simulink model "stuSimulation"  (R2019b)
settings: Solver=VariableStepAuto  StartTime=0.0  StopTime=0.1  RelTol=1e-3
undefined symbols (not defined in the file): doppler
libraries: commchan3 x2, dspsrcs4 x2, dsparch4 x1
settings Model: Creator=dm  LastModifiedBy=LYM
settings DebuggingCC: SFMachineParentedDataDiag=error
settings GRTTargetCC: RTWCAPISignals=on  RTWCAPIParams=on

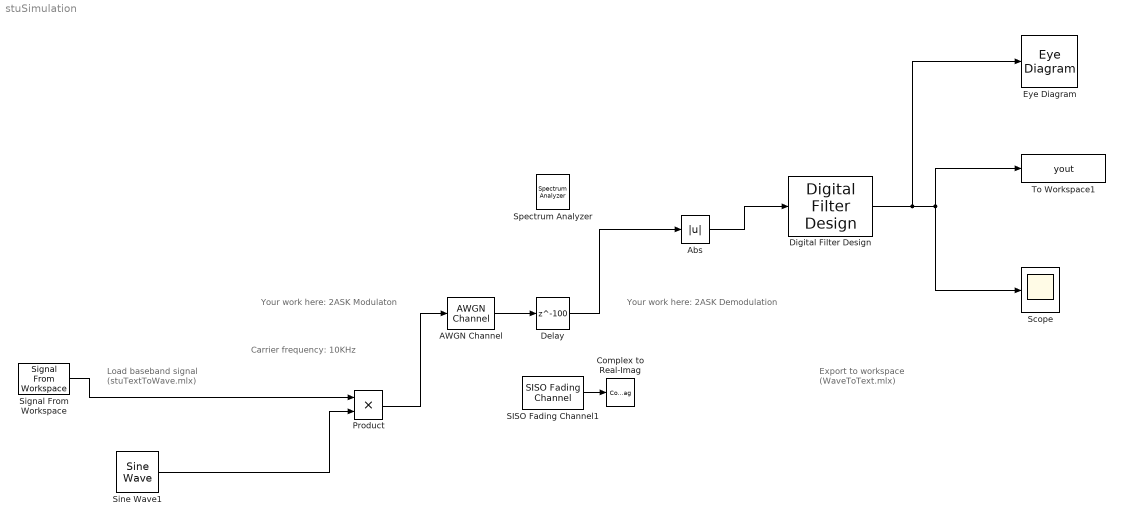
== system stuSimulation ==
  note: Load baseband signal
      | (stuTextToWave.mlx)
  note: Your work here:
      | 2ASK Modulaton
  note: Your work here:
      | 2ASK Demodulation
  note: Export to workspace
      | (WaveToText.mlx)
  note: Carrier frequency: 10KHz
  AWGN Channel : commchan3/AWGN Channel  InputProcessing=Columns as channels (frame based)  seed=67  noiseMode="Signal to noise ratio  (Eb/No)"  EbNodB=10  EsNodB=10  SNRdB=10  bitsPerSym=1  Ps=1e-3  Tsym=1e-3  variance=1
      settings: SourceProductName=Communications Toolbox
  Abs : Abs
  Complex to Real-Imag : ComplexToRealImag  Output=Real
  Delay : Delay  DelayLength=100  InputProcessing=Columns as channels (frame based)
  Digital Filter Design : dsparch4/Digital Filter Design  mwdsp_browser_bugfix_var=off
  Eye Diagram : EyeDiagram
  Product : Product
  SISO Fading Channel1 : commchan3/SISO Fading Channel  InheritSampleRate=on  SampleRate=1  PathDelays=0.001  AveragePathGains=-20  NormalizePathGains=on  FadingDistribution=Rician  KFactor=3  DirectPathDopplerShift=1  DirectPathInitialPhase=1  MaximumDopplerShift=2  DopplerSpectrum=doppler('Jakes')  RandomStream=mt19937ar with seed  Seed=73  PathGainsOutputPort=off  ChannelFilterDelayOutputPort=off  SimulateUsing=Interpreted execution  Visualization=Off  PathsForDopplerDisplay=1  SamplesToDisplay=25%
      settings: SourceProductName=Communications Toolbox
  Scope : Scope
  Signal From Workspace : dspsrcs4/Signal From Workspace  X=txWave  Ts=1e-5  nsamps=1e4  OutputAfterFinalValue=Cyclic repetition  ignoreOrWarnInputAndFrameLengths=off  OutputFrames=off
  Sine Wave1 : dspsrcs4/Sine Wave  Amplitude=50  Frequency=10000  Phase=0  SampleMode=Discrete  OutComplex=Real  CompMethod=Trigonometric fcn  TableSize=Speed  SampleTime=1e-5  SamplesPerFrame=1e4  ResetState=Catch up to simulation time  OutputFrames=off  dataType=double  wordLen=16  udDataType=sfix(16)  fracBitsMode=Best precision  numFracBits=15  OutDataTypeStr=double  LastOutDataTypeStr=double
  Spectrum Analyzer : SpectrumAnalyzer
  To Workspace1 : ToWorkspace  VariableName=yout  SampleTime=1e-5
      settings: MaxDataPoints=1e5  Decimation=1e4  Save2DSignal=2-D array (concatenate along first dimension)
  wires:
  Sine Wave1/1 -> Product/2
  Signal From Workspace/1 -> Product/1
  Abs/1 -> Digital Filter Design/1
  Digital Filter Design/1 -> Eye Diagram/1, Scope/1, To Workspace1/1
  SISO Fading Channel1/1 -> Complex to Real-Imag/1
  AWGN Channel/1 -> Delay/1
  Product/1 -> AWGN Channel/1
  Delay/1 -> Abs/1
